simulink model "T15_DD1"  (R2016b)
settings: configuration reference "CodeGenConfigSet" (kept outside this file)
values from neighbouring files (symbols this model uses):
  T15_tiDebHiLo_C = Calibration.Parameter    [init_T15_DD.m]
  T15_tiDebLoHi_C = Calibration.Parameter    [init_T15_DD.m]
  T15_uThreshold_C = Calibration.Parameter    [init_T15_DD.m]
undefined symbols (not defined in the file or in its folder): T15_DD_DT
libraries: CXLib x1
settings Model: Creator=Administrator  LastModifiedBy=Administrator
settings ConfigSetRef: SourceLocation=Base Workspace

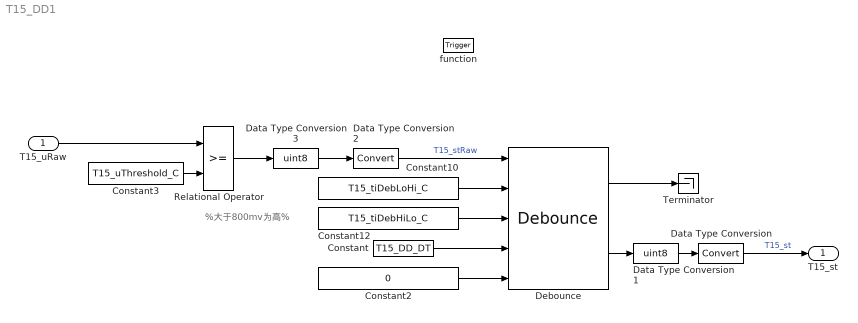
== system T15_DD1 ==
  note: %大于800mv为高%
  T15_uRaw : Inport  Tag=mv  Description=Raw ADC value of downstream engine coolant temperature sensor signal  OutMin=0  OutMax=5000  OutDataTypeStr=Ad_mv
  function : TriggerPort  TriggerType=function-call  VariantControl=Variant
  Constant : Constant  Value=T15_DD_DT
  Constant10 : Constant  Value=T15_tiDebLoHi_C
  Constant12 : Constant  Value=T15_tiDebHiLo_C
  Constant2 : Constant  Value=0  OutDataTypeStr=boolean
  Constant3 : Constant  Value=T15_uThreshold_C
  Data Type Conversion : DataTypeConversion
  Data Type Conversion1 : DataTypeConversion  OutDataTypeStr=uint8
  Data Type Conversion2 : DataTypeConversion
  Data Type Conversion3 : DataTypeConversion  OutDataTypeStr=uint8
  Debounce : CXLib/Debounce
  Relational Operator : RelationalOperator  OutDataTypeStr=boolean  RndMeth=Nearest  InputSameDT=on
  Terminator : Terminator
  T15_st : Outport  Description=Terminal 15 status after debouncing  OutDataTypeStr=Enum: Switch_conv
  wires:
  Debounce/2 -> Data Type Conversion1/1
  Constant10/1 -> Debounce/2
  Constant12/1 -> Debounce/3
  Constant/1 -> Debounce/4
  Constant2/1 -> Debounce/5
  Debounce/1 -> Terminator/1
  Data Type Conversion/1 -> T15_st/1  "T15_st"
  Data Type Conversion1/1 -> Data Type Conversion/1
  T15_uRaw/1 -> Relational Operator/1
  Relational Operator/1 -> Data Type Conversion3/1
  Data Type Conversion2/1 -> Debounce/1  "T15_stRaw"
  Data Type Conversion3/1 -> Data Type Conversion2/1
  Constant3/1 -> Relational Operator/2
